simulink model "x1_SimpleShaft"  (R2023a)
settings: Solver=ode1  StartTime=0.0  StopTime=10.0  FixedStep=0.02  RelTol=1e-3
values from neighbouring files (symbols this model uses):
  b = 1    [x1_init1.m]
  const_torque = 1    [x1_init1.m]
  J = 1    [x1_init1.m]
  omega0 = 0    [x1_init1.m]
  theta0 = 0    [x1_init1.m]
settings Model: Creator=sgopalswamy  LastModifiedBy=swami
settings SolverCC: AlgebraicLoopSolver=TrustRegion
settings DataIOCC: ReturnWorkspaceOutputs=off
settings DebuggingCC: UnconnectedInputMsg=warning  UnconnectedOutputMsg=warning  UnconnectedLineMsg=warning  ArithmeticOperatorsInVariantConditions=warning
settings ModelReferenceCC: EnableRefExpFcnMdlSchedulingChecks=on
settings SFSimCC: SimUseLocalCustomCode=off  CustomCodeUndefinedFunction=UseInterfaceOnly
settings RTWCC: RTWUseLocalCustomCode=off
settings CodeAppCC: StateflowObjectComments=on

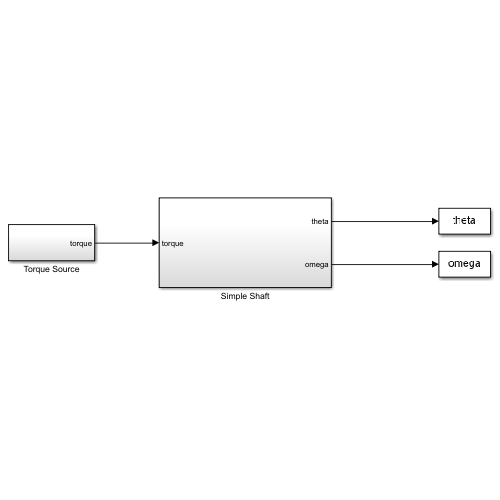
[thumbnail: Simulink's stored preview of the top-level diagram]
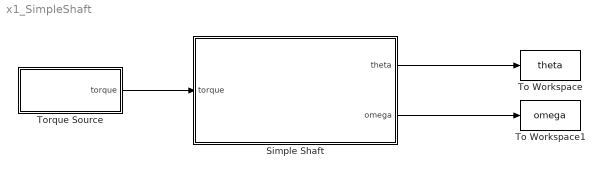
== system x1_SimpleShaft ==
  Simple Shaft : Subsystem
  To Workspace : ToWorkspace  VariableName=theta  SaveFormat=Timeseries  SampleTime=-1
  To Workspace1 : ToWorkspace  VariableName=omega  SaveFormat=Timeseries  SampleTime=-1
  Torque Source : Subsystem
  wires:
  Torque Source/1(torque) -> Simple Shaft/1(torque)
  Simple Shaft/1(theta) -> To Workspace/1
  Simple Shaft/2(omega) -> To Workspace1/1

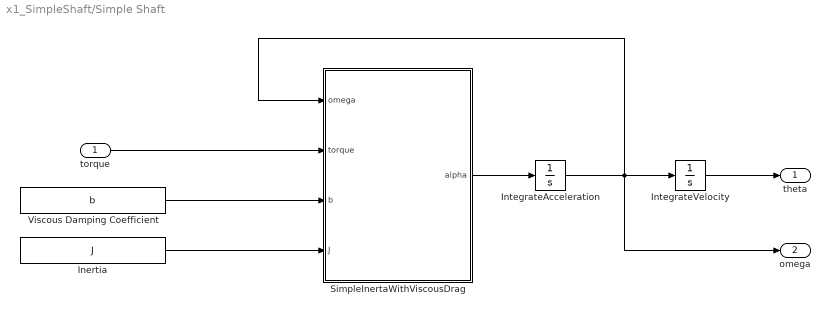
== system x1_SimpleShaft/Simple Shaft ==
  torque : Inport
  Inertia : Constant  Value=J
  IntegrateAcceleration : Integrator  InitialCondition=omega0
  IntegrateVelocity : Integrator  InitialCondition=theta0
  SimpleInertaWithViscousDrag : MATLAB Function  TreatAsAtomicUnit=on
  Viscous Damping Coefficient : Constant  Value=b
  theta : Outport
  omega : Outport  Port=2
  wires:
  IntegrateAcceleration/1 -> omega/1, SimpleInertaWithViscousDrag/1(omega), IntegrateVelocity/1
  IntegrateVelocity/1 -> theta/1
  SimpleInertaWithViscousDrag/1(alpha) -> IntegrateAcceleration/1
  torque/1 -> SimpleInertaWithViscousDrag/2(torque)
  Viscous Damping Coefficient/1 -> SimpleInertaWithViscousDrag/3(b)
  Inertia/1 -> SimpleInertaWithViscousDrag/4(J)

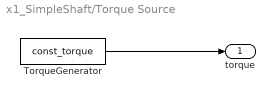
== system x1_SimpleShaft/Torque Source ==
  TorqueGenerator : Constant  Value=const_torque
  torque : Outport
  wires:
  TorqueGenerator/1 -> torque/1

== matlab function x1_SimpleShaft/Simple Shaft/SimpleInertaWithViscousDrag ==
  data: omega input; torque input; alpha output; b input; J input
function alpha = fcn(omega, torque,b, J)
alpha = (torque - omega * b)/J;
